simulink model "testDisc"  (Simulink 7.9)
settings: Solver=ode45  StartTime=0.0  StopTime=10.0  RelTol=1e-3
values from neighbouring files (symbols this model uses):
  AD = TT*AD*inv(TT)    [tuneXYControl.m]
  BD = TT*BD    [tuneXYControl.m]
  delay = delay + 0.14    (= 0.34)    [tuneXYControl.m]
  sampleTs = 0.2    [tuneXYControl.m]
  ssc = ss(tfc)    [tuneXYControl.m]
  sscaccel = ss(tfcaccel)    [tuneXYControl.m]
  sscvel = ss(tfcvel)    [tuneXYControl.m]
settings Model: Creator=user  LastModifiedBy=user

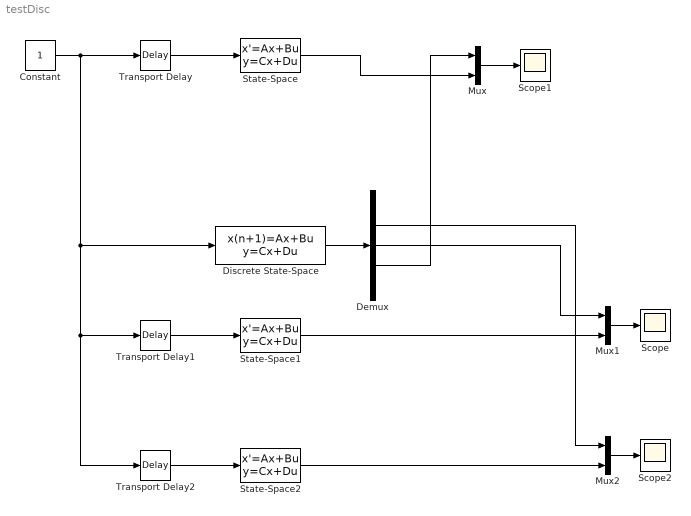
== system testDisc ==
  Constant : Constant
  Demux : Demux  Outputs=length(AD)
  Discrete State-Space : DiscreteStateSpace  A=AD  B=BD  C=eye(length(AD))  D=zeros(length(AD),1)  SampleTime=sampleTs
  Mux : Mux  Inputs=2
  Mux1 : Mux  Inputs=2
  Mux2 : Mux  Inputs=2
  Scope : Scope
  Scope1 : Scope
  Scope2 : Scope
      settings: SaveName=ScopeData2
  State-Space : StateSpace  A=ssc.a  B=ssc.b  C=ssc.c  D=ssc.d
  State-Space1 : StateSpace  A=sscvel.a  B=sscvel.b  C=sscvel.c  D=sscvel.d
  State-Space2 : StateSpace  A=sscaccel.a  B=sscaccel.b  C=sscaccel.c  D=sscaccel.d
  Transport Delay : TransportDelay  DelayTime=delay
  Transport Delay1 : TransportDelay  DelayTime=delay
  Transport Delay2 : TransportDelay  DelayTime=delay
  wires:
  Constant/1 -> Transport Delay/1, Discrete State-Space/1, Transport Delay1/1, Transport Delay2/1
  Transport Delay/1 -> State-Space/1
  State-Space/1 -> Mux/2
  Discrete State-Space/1 -> Demux/1
  Demux/3 -> Mux1/1
  Demux/4 -> Mux/1
  Demux/2 -> Mux2/1
  State-Space2/1 -> Mux2/2
  Mux/1 -> Scope1/1
  Mux1/1 -> Scope/1
  Mux2/1 -> Scope2/1
  State-Space1/1 -> Mux1/2
  Transport Delay1/1 -> State-Space1/1
  Transport Delay2/1 -> State-Space2/1
